simulink model "practica_411"  (Simulink 5.0)
settings: Solver=ode45  StartTime=0.0  StopTime=100.0  RelTol=1e-3
undefined symbols (not defined in the file): ts
libraries: dspmtrx3 x8, simulink x3, dspinverses x1
settings Model: LastModifiedBy=LeO

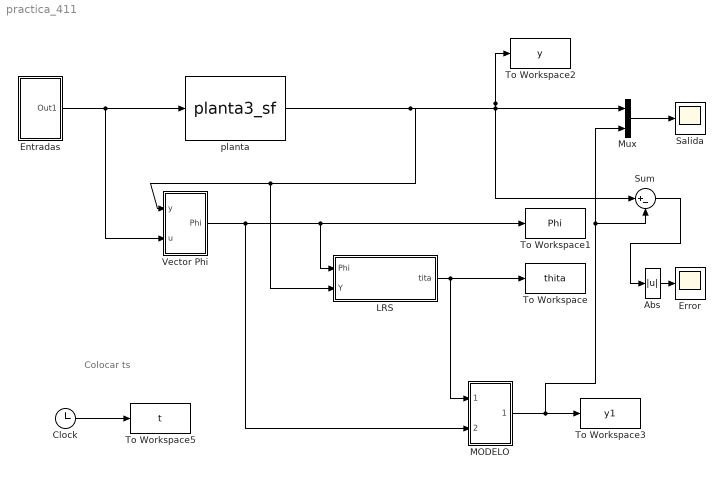
== system practica_411 ==
  note: Colocar ts
  Abs : Abs  SaturateOnIntegerOverflow=on
  Clock : Clock
      settings: Decimation=10
  Entradas : Subsystem
  Error : Scope
  LRS : Subsystem
  MODELO : Subsystem
  Mux : Mux  Inputs=2
  Salida : Scope
  Sum : Sum  Inputs=|+-  SaturateOnIntegerOverflow=on
  To Workspace : ToWorkspace  VariableName=thita  SampleTime=ts  SaveFormat=Array
  To Workspace1 : ToWorkspace  VariableName=Phi  SampleTime=ts  SaveFormat=Array
  To Workspace2 : ToWorkspace  VariableName=y  SampleTime=ts  SaveFormat=Array
  To Workspace3 : ToWorkspace  VariableName=y1  SampleTime=ts  SaveFormat=Array
  To Workspace5 : ToWorkspace  VariableName=t  SampleTime=ts  SaveFormat=Array
  Vector Phi : Subsystem
  planta : S-Function  FunctionName=planta3_sf
  wires:
  Vector Phi/1(Phi) -> LRS/1("Phi "), To Workspace1/1, MODELO/2(Phi)
  planta/1 -> Vector Phi/1("y "), LRS/2(Y), Mux/1, To Workspace2/1, Sum/1
  Entradas/1(Out1) -> planta/1, Vector Phi/2(u)
  LRS/1(tita) -> To Workspace/1, MODELO/1(thita)
  Clock/1 -> To Workspace5/1
  MODELO/1(Out1) -> To Workspace3/1, Mux/2, Sum/2
  Mux/1 -> Salida/1
  Sum/1 -> Abs/1
  Abs/1 -> Error/1

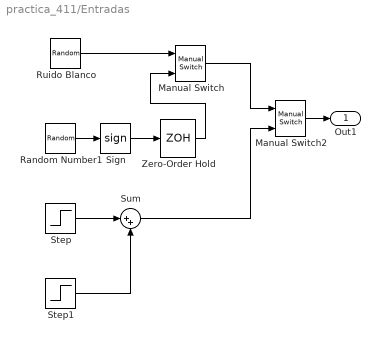
== system practica_411/Entradas ==
  Manual Switch : simulink/Signal Routing/Manual Switch  sw=0  action=0
  Manual Switch2 : simulink/Signal Routing/Manual Switch  sw=1  action=0
  Random Number1 : RandomNumber  SampleTime=0
  Ruido Blanco : RandomNumber  Variance=20  Seed=12  SampleTime=ts
  Sign : Signum
  Step : Step  Time=2  After=5  SampleTime=0.05
  Step1 : Step  Time=20  After=20  SampleTime=0.05
  Sum : Sum  Inputs=|++  SaturateOnIntegerOverflow=on
  Zero-Order Hold : ZeroOrderHold  SampleTime=0.05
  Out1 : Outport
  wires:
  Sign/1 -> Zero-Order Hold/1
  Random Number1/1 -> Sign/1
  Manual Switch/1 -> Manual Switch2/1
  Ruido Blanco/1 -> Manual Switch/1
  Zero-Order Hold/1 -> Manual Switch/2
  Sum/1 -> Manual Switch2/2
  Manual Switch2/1 -> Out1/1
  Step/1 -> Sum/1
  Step1/1 -> Sum/2

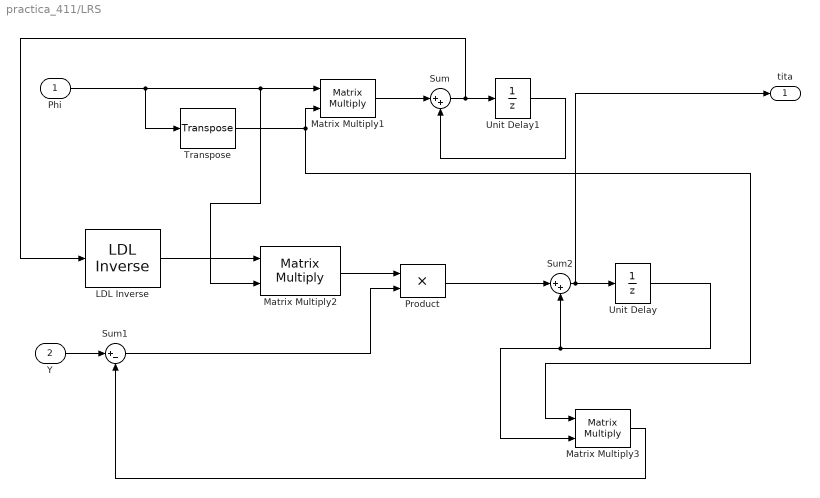
== system practica_411/LRS ==
  "Phi " : Inport  SampleTime=ts
  Y : Inport  Port=2  SampleTime=ts
  LDL Inverse : dspinverses/LDL Inverse  errmode=Ignore
  Matrix Multiply1 : dspmtrx3/Matrix Multiply  numInputPorts=2  OptimizationLevel=None
  Matrix Multiply2 : dspmtrx3/Matrix Multiply  numInputPorts=2  OptimizationLevel=None
  Matrix Multiply3 : dspmtrx3/Matrix Multiply  numInputPorts=2  OptimizationLevel=None
  Product : Product  SaturateOnIntegerOverflow=on
  Sum : Sum  Inputs=|++  SaturateOnIntegerOverflow=on
  Sum1 : Sum  Inputs=|+-  SaturateOnIntegerOverflow=on
  Sum2 : Sum  Inputs=|++  SaturateOnIntegerOverflow=on
  Transpose : dspmtrx3/Transpose  Hermitian=off
  Unit Delay : UnitDelay  X0=1*10^-3  SampleTime=ts
  Unit Delay1 : UnitDelay  X0=10^-3  SampleTime=ts
  tita : Outport
  wires:
  "Phi "/1 -> Transpose/1, Matrix Multiply1/1, Matrix Multiply2/2
  Transpose/1 -> Matrix Multiply1/2, Matrix Multiply3/1
  Matrix Multiply1/1 -> Sum/1
  Sum/1 -> Unit Delay1/1, LDL Inverse/1
  Unit Delay1/1 -> Sum/2
  LDL Inverse/1 -> Matrix Multiply2/1
  Sum2/1 -> Unit Delay/1, tita/1
  Y/1 -> Sum1/1
  Matrix Multiply2/1 -> Product/1
  Product/1 -> Sum2/1
  Matrix Multiply3/1 -> Sum1/2
  Sum1/1 -> Product/2
  Unit Delay/1 -> Matrix Multiply3/2, Sum2/2

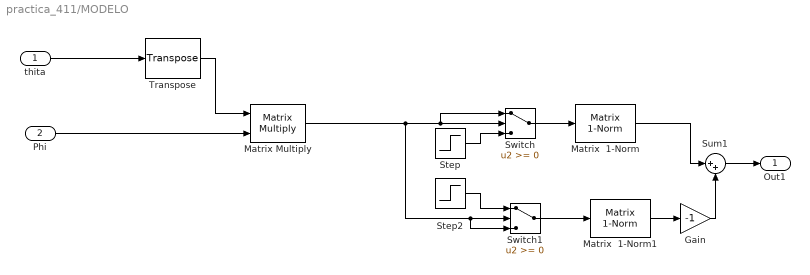
== system practica_411/MODELO ==
  thita : Inport
  Phi : Inport  Port=2
  Gain : Gain  Gain=-1  SaturateOnIntegerOverflow=on
  Matrix  1-Norm : dspmtrx3/Matrix  1-Norm
  Matrix  1-Norm1 : dspmtrx3/Matrix  1-Norm
  Matrix Multiply : dspmtrx3/Matrix Multiply  numInputPorts=2  OptimizationLevel=None
  Step : Step  Time=0  After=0  SampleTime=0
  Step2 : Step  Time=0  After=0  SampleTime=0
  Sum1 : Sum  Inputs=|++  SaturateOnIntegerOverflow=on
  Switch : Switch  SaturateOnIntegerOverflow=on
  Switch1 : Switch  SaturateOnIntegerOverflow=on
  Transpose : dspmtrx3/Transpose  Hermitian=off
  Out1 : Outport
  wires:
  Phi/1 -> Matrix Multiply/2
  Transpose/1 -> Matrix Multiply/1
  thita/1 -> Transpose/1
  Matrix Multiply/1 -> Switch/2, Switch/1, Switch1/2, Switch1/3
  Sum1/1 -> Out1/1
  Step/1 -> Switch/3
  Switch/1 -> Matrix  1-Norm/1
  Switch1/1 -> Matrix  1-Norm1/1
  Step2/1 -> Switch1/1
  Matrix  1-Norm/1 -> Sum1/1
  Matrix  1-Norm1/1 -> Gain/1
  Gain/1 -> Sum1/2

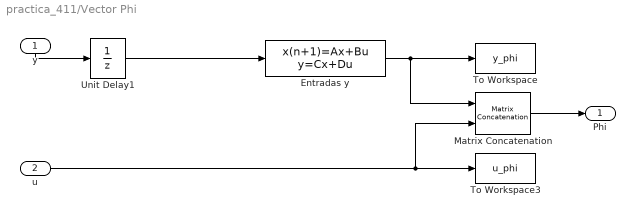
== system practica_411/Vector Phi ==
  "y " : Inport  Orientation=down  SampleTime=ts
  u : Inport  Port=2  SampleTime=ts
  Entradas y : DiscreteStateSpace  A=[0 0 0 0; 1 0 0 0; 0 1 0 0; 0 0 1 0]  B=[-1; 0; 0;0]  C=[eye(4)]  D=[0;0;0;0]  SampleTime=ts
  Matrix Concatenation : simulink/Math Operations/Matrix Concatenation  numInports=2  catMethod=Vertical
  To Workspace : ToWorkspace  VariableName=y_phi  SampleTime=ts  SaveFormat=Array
  To Workspace3 : ToWorkspace  VariableName=u_phi  SampleTime=ts  SaveFormat=Array
  Unit Delay1 : UnitDelay  SampleTime=ts
  Phi : Outport
  wires:
  Entradas y/1 -> To Workspace/1, Matrix Concatenation/1
  u/1 -> To Workspace3/1, Matrix Concatenation/2
  Matrix Concatenation/1 -> Phi/1
  "y "/1 -> Unit Delay1/1
  Unit Delay1/1 -> Entradas y/1
